simulink model "Simulacion_Temporal"  (R2023b)
settings: Solver=VariableStepAuto  StartTime=0.0  StopTime=1.9  FixedStep=1e-5  RelTol=1e-3
values from neighbouring files (symbols this model uses):
  P_p = 3    [diagrama_polos_y_ceros_LTI.m]    (also in main.m; parametros.m; variacion_de_parametros.m)
libraries: SignalEditorBlockLib x2
settings Model: Creator=Julya  LastModifiedBy=Julya
settings ModelReferenceCC: ModelReferenceMinAlgLoopOccurrences=on

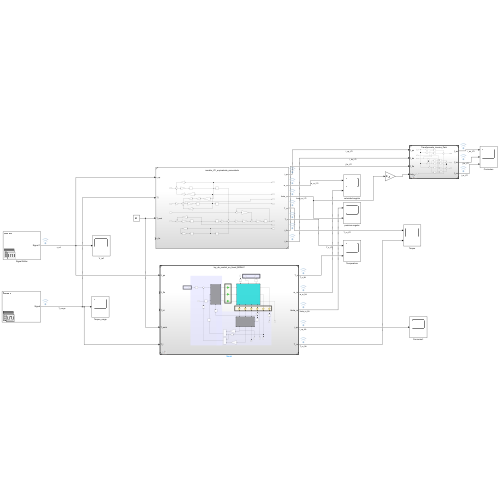
[thumbnail: Simulink's stored preview of the top-level diagram]
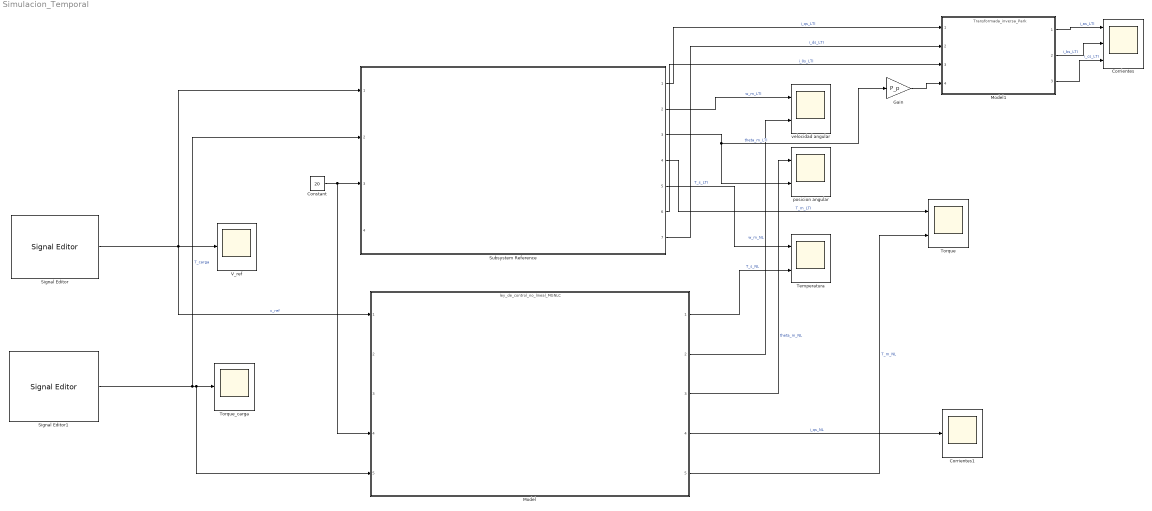
== system Simulacion_Temporal ==
  Constant : Constant  Value=20
  Corrientes : Scope  NumInputPorts=3
  Corrientes1 : Scope
  Gain : Gain  Gain=P_p
  Model : ModelReference  ModelNameDialog=ley_de_control_no_lineal_MGNLC.slx  SimulationMode=Normal  ModelReferenceVersion=1.31
  Model1 : ModelReference  ModelNameDialog=Transformada_inversa_Park.slx  SimulationMode=Normal  ModelReferenceVersion=1.5
  Signal Editor : SignalEditorBlockLib/Signal Editor  FileName=V_qs_ref.mat  ActiveScenario=Scenario  ActiveSignal=Signal 1  IsBus=off  OutputBusObjectStr=Bus: BusObject  SampleTime=0  Interpolate=off  ZeroCross=off  OutputAfterFinalValue=Setting to zero  Unit=inherit  PreserveSignalName=on  ApplySigPropsToAllScenarios=on  ApplySigPropsToAllSignals=off
  Signal Editor1 : SignalEditorBlockLib/Signal Editor  FileName=Pulso_Torque_Carga.mat  ActiveScenario=Scenario  ActiveSignal=Signal  IsBus=off  OutputBusObjectStr=Bus: BusObject  SampleTime=0  Interpolate=off  ZeroCross=off  OutputAfterFinalValue=Setting to zero  Unit=inherit  PreserveSignalName=on  ApplySigPropsToAllScenarios=on  ApplySigPropsToAllSignals=off
  Subsystem Reference : Subsystem  ReferencedSubsystem=modelo_LTI_equivalente_aumentado
  Temperatura : Scope  NumInputPorts=2
  Torque : Scope  NumInputPorts=2
  Torque_carga : Scope
  V_ref : Scope
  posicion angular : Scope  NumInputPorts=2
  velocidad angular : Scope  NumInputPorts=2
  wires:
  Signal Editor/1 -> Model/1, Subsystem Reference/1, V_ref/1  "v_ref"
  Subsystem Reference/1 -> Model1/1  "i_qs_LTI"
  Subsystem Reference/2 -> velocidad angular/1  "w_m_LTI"
  Subsystem Reference/3 -> Gain/1, posicion angular/2  "theta_m_LTI"
  Subsystem Reference/5 -> Temperatura/1  "T_s_LTI"
  Signal Editor1/1 -> Subsystem Reference/2, Model/5, Torque_carga/1  "T_carga"
  Constant/1 -> Model/4, Subsystem Reference/3
  Subsystem Reference/4 -> Torque/1  "T_m_LTI"
  Model/1 -> Temperatura/2  "T_s_NL"
  Model/2 -> velocidad angular/2  "w_m_NL"
  Model/3 -> posicion angular/1  "theta_m_NL"
  Model/5 -> Torque/2  "T_m_NL"
  Subsystem Reference/6 -> Model1/3  "i_0s_LTI"
  Subsystem Reference/7 -> Model1/2  "i_ds_LTI"
  Gain/1 -> Model1/4
  Model1/1 -> Corrientes/1  "i_as_LTI"
  Model1/2 -> Corrientes/2  "i_bs_LTI"
  Model1/3 -> Corrientes/3  "i_cs_LTI"
  Model/4 -> Corrientes1/1  "i_qs_NL"
